simulink model "numerical_simulation_without_controller"  (R2015b)
settings: Solver=VariableStepAuto  StartTime=0.0  StopTime=5  RelTol=1e-3
values from neighbouring files (symbols this model uses):
  A0 = 0    [Initial_Conditions.m]
  Bh = block.DialogPrm(2).Data    [HapticDevice.m]    (also in Initial_Conditions.m = 3.62)
  Bo = block.DialogPrm(2).Data    [HumanOperator.m]    (also in Initial_Conditions.m = 5.5)
  BWall = 0    [Initial_Conditions.m]
  Ffriction = block.DialogPrm(1).Data    [HapticDevice.m]    (also in Initial_Conditions.m = 0.024)
  Ko = block.DialogPrm(3).Data    [HumanOperator.m]    (also in Initial_Conditions.m = 30)
  KWall = 10000    [Initial_Conditions.m]
  Mh = block.DialogPrm(3).Data    [HapticDevice.m]    (also in Initial_Conditions.m = 0.032)
  Mo = block.DialogPrm(1).Data    [HumanOperator.m]    (also in Initial_Conditions.m = 0.8)
  nWall = block.DialogPrm(6).Data    [Controller1.m]    (also in HapticController.m = block.DialogPrm(3).Data; Initial_Conditions.m = -1; Initiation.m = -1; MoreConservative.m = block.DialogPrm(5).Data)
  tinterval = block.DialogPrm(4).Data    [HapticDevice.m]    (also in HumanOperator.m = block.DialogPrm(8).Data; Initial_Conditions.m = 1e-05)
  tsampling = block.DialogPrm(3).Data    [Controller.m]    (also in Controller1.m; Controller_more.m = block.DialogPrm(4).Data; HapticController.m = block.DialogPrm(6).Data; Initial_Conditions.m = 0.001)
  V0 = 0    [Initial_Conditions.m]
  X0 = 0    [Initial_Conditions.m]
  Xeq = block.DialogPrm(4).Data    [HumanOperator.m]    (also in Initial_Conditions.m = 0.08)
  XWall = 0.04    [Initial_Conditions.m]
libraries: simulink x2
settings Model: Creator=TOSHIBA  LastModifiedBy=TOSHIBA

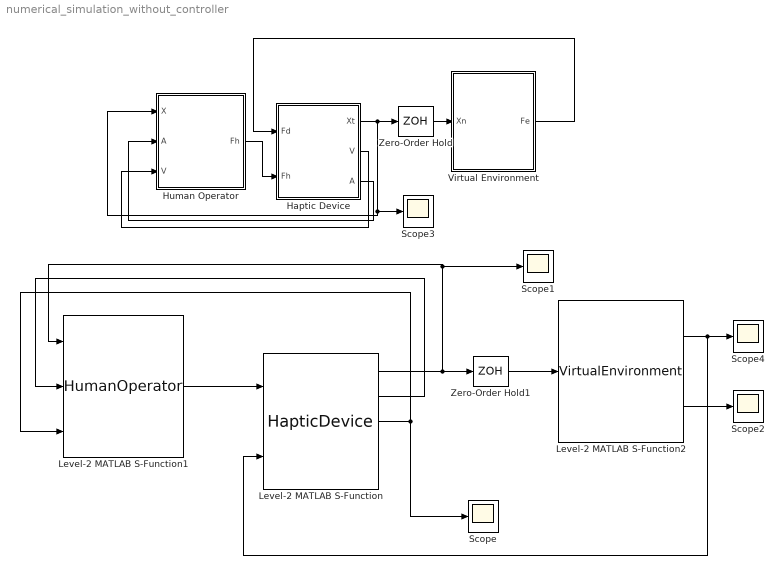
== system numerical_simulation_without_controller ==
  Haptic Device : Subsystem
  Human Operator : Subsystem
  Level-2 MATLAB S-Function : M-S-Function  FunctionName=HapticDevice  Parameters=Ffriction,Bh,Mh,tinterval,X0,V0
  Level-2 MATLAB S-Function1 : M-S-Function  FunctionName=HumanOperator  Parameters=Mo,Bo,Ko,Xeq,X0,V0,A0,tinterval
  Level-2 MATLAB S-Function2 : M-S-Function  FunctionName=VirtualEnvironment  Parameters=KWall,BWall,nWall,XWall,tsampling
  Scope{,1..4} (5 alike) : Scope
  Virtual Environment : Subsystem
  Zero-Order Hold : ZeroOrderHold  SampleTime=tsampling
  Zero-Order Hold1 : ZeroOrderHold  SampleTime=tsampling
  wires:
  Haptic Device/1(Xt) -> Scope3/1, Human Operator/1(X), Zero-Order Hold/1
  Zero-Order Hold/1 -> Virtual Environment/1(Xn)
  Human Operator/1(Fh) -> Haptic Device/2(Fh)
  Haptic Device/2(V) -> Human Operator/3(V)
  Haptic Device/3(A) -> Human Operator/2(A)
  Level-2 MATLAB S-Function/3 -> Level-2 MATLAB S-Function1/3, Scope/1
  Level-2 MATLAB S-Function/1 -> Level-2 MATLAB S-Function1/1, Scope1/1, Zero-Order Hold1/1
  Level-2 MATLAB S-Function/2 -> Level-2 MATLAB S-Function1/2
  Level-2 MATLAB S-Function1/1 -> Level-2 MATLAB S-Function/1
  Level-2 MATLAB S-Function2/2 -> Scope2/1
  Level-2 MATLAB S-Function2/1 -> Level-2 MATLAB S-Function/2, Scope4/1
  Virtual Environment/1(Fe) -> Haptic Device/1(Fd)
  Zero-Order Hold1/1 -> Level-2 MATLAB S-Function2/1

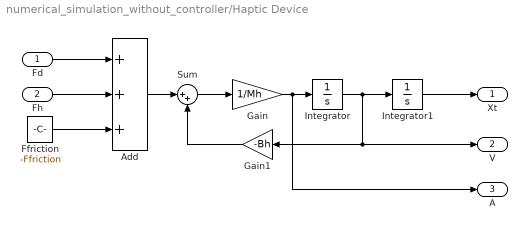
== system numerical_simulation_without_controller/Haptic Device ==
  Fd : Inport
  Fh : Inport  Port=2
  Add : Sum  Inputs=+++
  Ffriction : Constant  Value=-Ffriction
  Gain : Gain  Gain=1/Mh
  Gain1 : Gain  Gain=-Bh
  Integrator : Integrator  InitialCondition=V0
  Integrator1 : Integrator  InitialCondition=X0
  Sum : Sum  Inputs=|++
  Xt : Outport
  V : Outport  Port=2
  A : Outport  Port=3
  wires:
  Integrator/1 -> Integrator1/1, Gain1/1, V/1
  Gain/1 -> A/1, Integrator/1
  Integrator1/1 -> Xt/1
  Ffriction/1 -> Add/3
  Fh/1 -> Add/2
  Fd/1 -> Add/1
  Sum/1 -> Gain/1
  Gain1/1 -> Sum/2
  Add/1 -> Sum/1

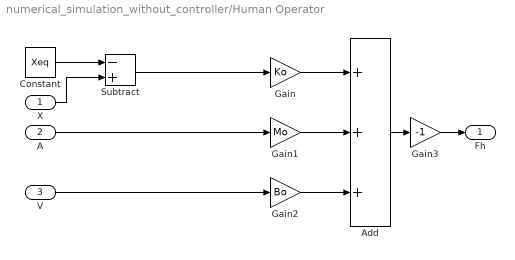
== system numerical_simulation_without_controller/Human Operator ==
  X : Inport
  A : Inport  Port=2
  V : Inport  Port=3
  Add : Sum  Inputs=+++
  Constant : Constant  Value=Xeq
  Gain : Gain  Gain=Ko
  Gain1 : Gain  Gain=Mo
  Gain2 : Gain  Gain=Bo
  Gain3 : Gain  Gain=-1
  Subtract : Sum  Inputs=-+
  Fh : Outport
  wires:
  X/1 -> Subtract/2
  Gain/1 -> Add/1
  Gain2/1 -> Add/3
  Constant/1 -> Subtract/1
  A/1 -> Gain1/1
  Subtract/1 -> Gain/1
  Add/1 -> Gain3/1
  Gain1/1 -> Add/2
  Gain3/1 -> Fh/1
  V/1 -> Gain2/1

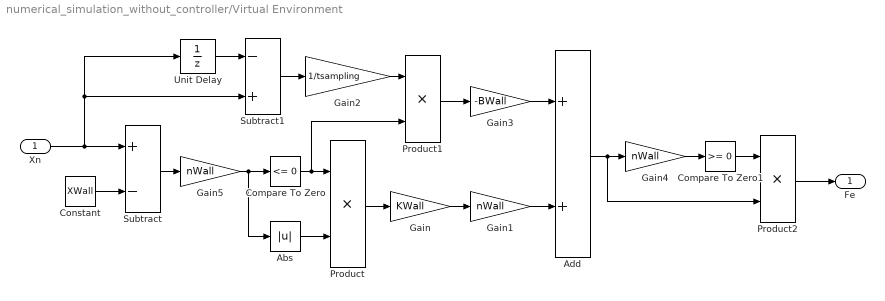
== system numerical_simulation_without_controller/Virtual Environment ==
  Xn : Inport
  Abs : Abs
  Add : Sum
  Compare To Zero : simulink/Logic and Bit Operations/Compare To Zero  relop=<=  OutDataTypeStr=boolean
  Compare To Zero1 : simulink/Logic and Bit Operations/Compare To Zero  relop=>=  OutDataTypeStr=boolean
  Constant : Constant  Value=XWall
  Gain : Gain  Gain=KWall
  Gain1 : Gain  Gain=nWall
  Gain2 : Gain  Gain=1/tsampling
  Gain3 : Gain  Gain=-BWall
  Gain4 : Gain  Gain=nWall
  Gain5 : Gain  Gain=nWall
  Product : Product
  Product1 : Product
  Product2 : Product
  Subtract : Sum  Inputs=+-
  Subtract1 : Sum  Inputs=-+
  Unit Delay : UnitDelay  InitialCondition=X0  SampleTime=tsampling
  Fe : Outport
  wires:
  Unit Delay/1 -> Subtract1/1
  Product/1 -> Gain/1
  Constant/1 -> Subtract/2
  Gain/1 -> Gain1/1
  Xn/1 -> Subtract/1, Subtract1/2, Unit Delay/1
  Abs/1 -> Product/2
  Compare To Zero/1 -> Product1/2, Product/1
  Product1/1 -> Gain3/1
  Gain3/1 -> Add/1
  Compare To Zero1/1 -> Product2/1
  Gain1/1 -> Add/2
  Subtract/1 -> Gain5/1
  Gain2/1 -> Product1/1
  Subtract1/1 -> Gain2/1
  Gain4/1 -> Compare To Zero1/1
  Add/1 -> Product2/2, Gain4/1
  Product2/1 -> Fe/1
  Gain5/1 -> Abs/1, Compare To Zero/1
